simulink model "battery_verification_model"  (R2024a)
settings: Solver=FixedStepAuto  StartTime=0.0  StopTime=10.0  RelTol=1e-3
libraries: dspsrcs4 x1
settings Model: Creator=fercl  LastModifiedBy=fercl

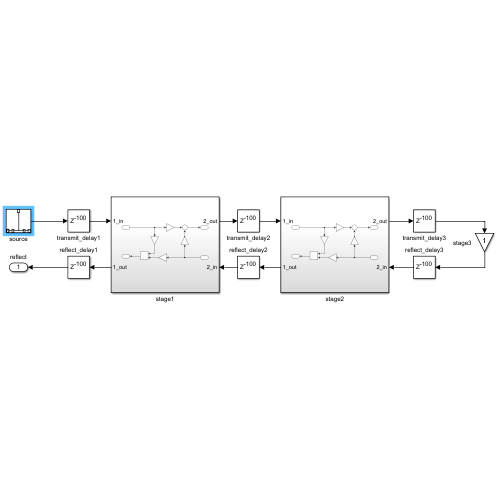
[thumbnail: Simulink's stored preview of the top-level diagram]
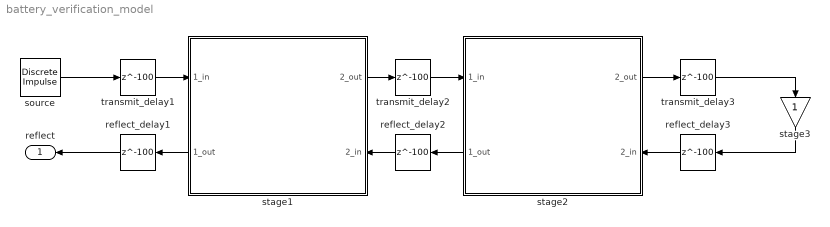
== system battery_verification_model ==
  reflect_delay1 : Delay  DelayLength=100  InputProcessing=Columns as channels (frame based)
  reflect_delay2 : Delay  DelayLength=100  InputProcessing=Columns as channels (frame based)
  reflect_delay3 : Delay  DelayLength=100  InputProcessing=Columns as channels (frame based)
  source : dspsrcs4/Discrete  Impulse  Delay=0  SampleTime=-1  FrameSample=1  OutputFrames=off  dataType=double  isSigned=on  wordLen=16  udDataType=sfix(16)  fracBitsMode=Best precision  numFracBits=15  OutDataTypeStr=double  LastOutDataTypeStr=double
  stage1 : Subsystem
      settings: PortSchema="{\"entries\":[{\"content\":{\"sides\":[{\"content\":{\"connectorIds\":[\"In1\",\"Out2\"]},\"type\":\"ConnectorPlacement.EquallySpacedRectSide\",\"uuid\":\"f88134b1-e3b7-4c65-b168-c6d4f3449b4f\"},{\"content\":{\"connectorIds\":[\"Out1\",\"In2\"],\"side\":\"RIGHT\"},\"type\":\"ConnectorPlacement.EquallySpacedRectSide\",\"uuid\":\"b9302cb7-b979-411c-93f3-70777302b38c\"},{\"content\":{\"side\":\"TOP\"},\"type\":\"ConnectorPlacement.EquallySpacedRectSide\",\"uuid\":\"07ce0f73-468e-4f30-9dbc-f1d98441728e\"}]},\"type\":\"ConnectorPlacement.EquallySpacedConnector\",\"uuid\":\"d8756f6c-ce1f-494d-91b0-49b8b171b11c\"}],\"packageUris\":[\"http://schema.mathworks.com/mf0/Connector/R2020b\"],\"version\":\"1.0\"}"
  stage2 : Subsystem
      settings: PortSchema="{\"entries\":[{\"content\":{\"sides\":[{\"content\":{\"connectorIds\":[\"In1\",\"Out2\"]},\"type\":\"ConnectorPlacement.EquallySpacedRectSide\",\"uuid\":\"f88134b1-e3b7-4c65-b168-c6d4f3449b4f\"},{\"content\":{\"connectorIds\":[\"Out1\",\"In2\"],\"side\":\"RIGHT\"},\"type\":\"ConnectorPlacement.EquallySpacedRectSide\",\"uuid\":\"b9302cb7-b979-411c-93f3-70777302b38c\"},{\"content\":{\"side\":\"TOP\"},\"type\":\"ConnectorPlacement.EquallySpacedRectSide\",\"uuid\":\"07ce0f73-468e-4f30-9dbc-f1d98441728e\"}]},\"type\":\"ConnectorPlacement.EquallySpacedConnector\",\"uuid\":\"d8756f6c-ce1f-494d-91b0-49b8b171b11c\"}],\"packageUris\":[\"http://schema.mathworks.com/mf0/Connector/R2020b\"],\"version\":\"1.0\"}"
  stage3 : Gain
  transmit_delay1 : Delay  DelayLength=100  InputProcessing=Columns as channels (frame based)
  transmit_delay2 : Delay  DelayLength=100  InputProcessing=Columns as channels (frame based)
  transmit_delay3 : Delay  DelayLength=100  InputProcessing=Columns as channels (frame based)
  reflect : Outport  OutDataTypeStr=double
  wires:
  reflect_delay1/1 -> reflect/1
  source/1 -> transmit_delay1/1
  stage3/1 -> reflect_delay3/1
  transmit_delay3/1 -> stage3/1
  transmit_delay1/1 -> stage1/1(1_in)
  stage1/1(2_out) -> transmit_delay2/1
  stage1/2(1_out) -> reflect_delay1/1
  reflect_delay2/1 -> stage1/2(2_in)
  transmit_delay2/1 -> stage2/1(1_in)
  stage2/2(1_out) -> reflect_delay2/1
  reflect_delay3/1 -> stage2/2(2_in)
  stage2/1(2_out) -> transmit_delay3/1

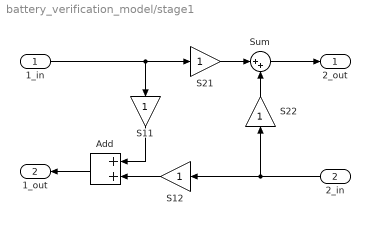
== system battery_verification_model/stage1 ==
  1_in : Inport  OutDataTypeStr=double
  2_in : Inport  Port=2
  Add : Sum
  S11 : Gain
  S12 : Gain
  S21 : Gain  OutDataTypeStr=double
  S22 : Gain
  Sum : Sum  Inputs=|++  OutDataTypeStr=double  AccumDataTypeStr=double
  2_out : Outport  OutDataTypeStr=double
  1_out : Outport  Port=2
  wires:
  S12/1 -> Add/2
  S11/1 -> Add/1
  S21/1 -> Sum/1
  Add/1 -> 1_out/1
  1_in/1 -> S11/1, S21/1
  S22/1 -> Sum/2
  2_in/1 -> S22/1, S12/1
  Sum/1 -> 2_out/1

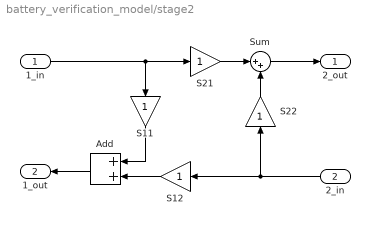
== system battery_verification_model/stage2 ==
  1_in : Inport
  2_in : Inport  Port=2
  Add : Sum
  S{11..12,21..22} (4 alike) : Gain
  Sum : Sum  Inputs=|++
  2_out : Outport
  1_out : Outport  Port=2
  wires:
  S12/1 -> Add/2
  S11/1 -> Add/1
  S21/1 -> Sum/1
  Add/1 -> 1_out/1
  1_in/1 -> S11/1, S21/1
  S22/1 -> Sum/2
  2_in/1 -> S22/1, S12/1
  Sum/1 -> 2_out/1
